simulink model "task_C1_mod_v2"  (R2018a)
settings: Solver=ode45  StartTime=0.0  StopTime=70  RelTol=1e-3  EnableMultiTasking=on
values from neighbouring files (symbols this model uses):
  a0 = 8*lamda/(c*ro*(b-a)^2)    [task_A_scr.m]    (also in task_B_scr.m = 8*lamda/(3*c*ro*(b-a)^2); task_C_scr.m = 4*lamda*(2-A1-B1)/(c*ro*(b-a)^2))
  A1 = x(1)    [task_C_scr.m]
  A2 = x(1)    [task_C_scr.m]
  A3 = x(1)    [task_C_scr.m]
  a_b = 30000    [task_C_scr.m]
  b1 = 4*lamda*(A2+B2)/(c*ro*(b-a)^2)    [task_C_scr.m]
  B1 = x(2)    [task_C_scr.m]
  b2 = 4*lamda*(A3+B3)/(c*ro*(b-a)^2)    [task_C_scr.m]
  B2 = x(2)    [task_C_scr.m]
  B3 = x(2)    [task_C_scr.m]
  c_b = 415    [task_C_scr.m]
  Q_b = 0.0425    [task_C_scr.m]
  ro_b = 1000    [task_C_scr.m]
  T_a = 350    [task_A_scr.m]    (also in task_C_scr.m = 600)
  T_b = 400    [task_A_scr.m]    (also in task_B_scr.m = 350; task_C_scr.m = 300)
undefined symbols (not defined in the file or in its folder): T_0
settings Model: Creator=Yurii  LastModifiedBy=Master
settings DataIOCC: LimitDataPoints=on  SaveFormat=Array
settings OptimizationCC: LifeSpan=inf
settings DebuggingCC: UnderspecifiedInitializationDetection=Classic  MergeDetectMultiDrivingBlocksExec=none  SolverPrmCheckMsg=warning  SFUnexpectedBacktrackingDiag=warning  SFNoUnconditionalDefaultTransitionDiag=warning  SFExecutionAtInitializationDiag=none
settings HardwareCC: ProdBitPerPointer=32  ProdBitPerSizeT=32  ProdBitPerPtrDiffT=32  ProdLargestAtomicFloat=None  ProdIntDivRoundTo=Undefined  ProdEndianess=Unspecified  ProdWordSize=32  ProdHWDeviceType=32-bit Generic
settings ModelReferenceCC: PropagateSignalLabelsOutOfModel=off
settings CodeAppCC: StateflowObjectComments=on
settings GRTTargetCC: TargetLangStandard=C89/C90 (ANSI)  GeneratePreprocessorConditionals=Disable all
settings ConfigComp: CovMetricSettings=dw  CovHtmlReporting=on  CovSaveCumulativeToWorkspaceVar=on  CovSaveSingleToWorkspaceVar=on  CovExternalEMLEnable=off

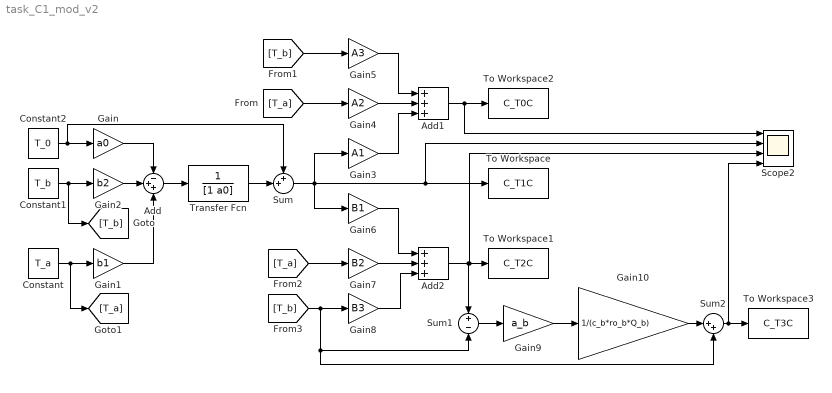
== system task_C1_mod_v2 ==
  Add : Sum  Inputs=-++
  Add1 : Sum  Inputs=+++
  Add2 : Sum  Inputs=+++
  Constant : Constant  Value=T_a
  Constant1 : Constant  Value=T_b
  Constant2 : Constant  Value=T_0
  Gain : Gain  Gain=a0
  Gain1 : Gain  Gain=b1
  Gain10 : Gain  Gain=1/(c_b*ro_b*Q_b)
  Gain2 : Gain  Gain=b2
  Gain3 : Gain  Gain=A1
  Gain4 : Gain  Gain=A2
  Gain5 : Gain  Gain=A3
  Gain6 : Gain  Gain=B1
  Gain7 : Gain  Gain=B2
  Gain8 : Gain  Gain=B3
  Gain9 : Gain  Gain=a_b
  Scope2 : Scope  NumInputPorts=4
  Sum : Sum  Inputs=++|
  Sum1 : Sum  Inputs=+|-
  Sum2 : Sum  Inputs=|++
  To Workspace : ToWorkspace  VariableName=C_T1C  SaveFormat=Timeseries  SampleTime=-1
  To Workspace1 : ToWorkspace  VariableName=C_T2C  SaveFormat=Timeseries  SampleTime=-1
  To Workspace2 : ToWorkspace  VariableName=C_T0C  SaveFormat=Timeseries  SampleTime=-1
  To Workspace3 : ToWorkspace  VariableName=C_T3C  SaveFormat=Timeseries  SampleTime=-1
  Transfer Fcn : TransferFcn  Denominator=[1 a0]
  wires:
  Constant1/1 -> [T_b], Gain2/1
  Constant2/1 -> Sum/1, Gain/1
  Gain/1 -> Add/1
  Add/1 -> Transfer Fcn/1
  Transfer Fcn/1 -> Sum/2
  Constant/1 -> [T_a], Gain1/1
  Gain1/1 -> Add/3
  Gain2/1 -> Add/2
  Sum/1 -> Gain6/1, Gain3/1, Scope2/2, To Workspace/1
  [T_a] -> Gain4/1
  [T_b] -> Gain5/1
  Gain4/1 -> Add1/2
  Gain5/1 -> Add1/1
  Gain3/1 -> Add1/3
  Add1/1 -> Scope2/1, To Workspace2/1
  [T_a] -> Gain7/1
  [T_b] -> Sum2/2, Sum1/2, Gain8/1
  Add2/1 -> Scope2/3, To Workspace1/1, Sum1/1
  Gain7/1 -> Add2/2
  Gain6/1 -> Add2/1
  Gain8/1 -> Add2/3
  Sum1/1 -> Gain9/1
  Gain9/1 -> Gain10/1
  Gain10/1 -> Sum2/1
  Sum2/1 -> Scope2/4, To Workspace3/1
